simulink model "DPTSpiceModel"  (R2016a)
settings: Solver=FixedStepDiscrete  StartTime=0.0  StopTime=0.55e-6  FixedStep=SampleTime  RelTol=1e-3
values from neighbouring files (symbols this model uses):
  Dbot = 48    [DPTSpiceMFile.m]    (also in LossCalcModelMFile.m = 49)
  DelayBot = 50    [DPTSpiceMFile.m]    (also in LossCalcModelMFile.m)
  DelayTop = 0    [DPTSpiceMFile.m]    (also in LossCalcModelMFile.m)
  Dtop = 48    [DPTSpiceMFile.m]    (also in LossCalcModelMFile.m = 49)
  fsw = 2000e3    (= 2000000)    [DPTSpiceMFile.m]    (also in LossCalcModelMFile.m = 1000000)
  InitialCurrent = LoadCurrent + CurrRipple/2    (= 30.1)    [DPTSpiceMFile.m]
  LoadCurrent = 30    [DPTSpiceMFile.m]
  Rd = 0.0024 + 1e-4    (= 0.0025)    [DPTSpiceMFile.m]    (also in LossCalcModelMFile.m = 2.5e-05; StepResponse.m)
  Rg = 1.5    [DPTSpiceMFile.m]    (also in LossCalcModelMFile.m; StepResponse.m)
  Roff = 2    [DPTSpiceMFile.m]    (also in LossCalcModelMFile.m = 5)
  Ron = 10    [DPTSpiceMFile.m]    (also in LossCalcModelMFile.m = 20)
  Rs = 0.0433 + 1e-4    (= 0.0434)    [DPTSpiceMFile.m]    (also in LossCalcModelMFile.m = 2.5e-05; StepResponse.m)
  Rss = 1e-3    (= 0.001)    [DPTSpiceMFile.m]    (also in StepResponse.m)
  SampleTime = 5e-13    [DPTSpiceMFile.m]    (also in LossCalcModelMFile.m)
  Vdc = 400    [DPTSpiceMFile.m]    (also in LossCalcModelMFile.m)
  VpulseMax = 6    [DPTSpiceMFile.m]    (also in LossCalcModelMFile.m; StepResponse.m)
  VpulseMin = -3    [DPTSpiceMFile.m]    (also in LossCalcModelMFile.m; StepResponse.m)
undefined symbols (not defined in the file or in its folder): DiscIntNeverNeededParam
libraries: elec_lib x50, nesl_utility x34, fl_lib x30, simulink x2
(part 1 of 2)
settings Model: Creator=ugurm  LastModifiedBy=kkfrk
settings OptimizationCC: EfficientMapNaN2IntZero=off
settings HardwareCC: TargetBitPerPointer=64  TargetLongLongMode=on  TargetIntDivRoundTo=Zero  TargetEndianess=LittleEndian  TargetWordSize=64  TargetHWDeviceType=MATLAB Host  ProdEqTarget=off
settings CodeAppCC: MaxIdLength=128
settings GRTTargetCC: GeneratePreprocessorConditionals=Use local settings  CombineOutputUpdateFcns=off  GRTInterface=on

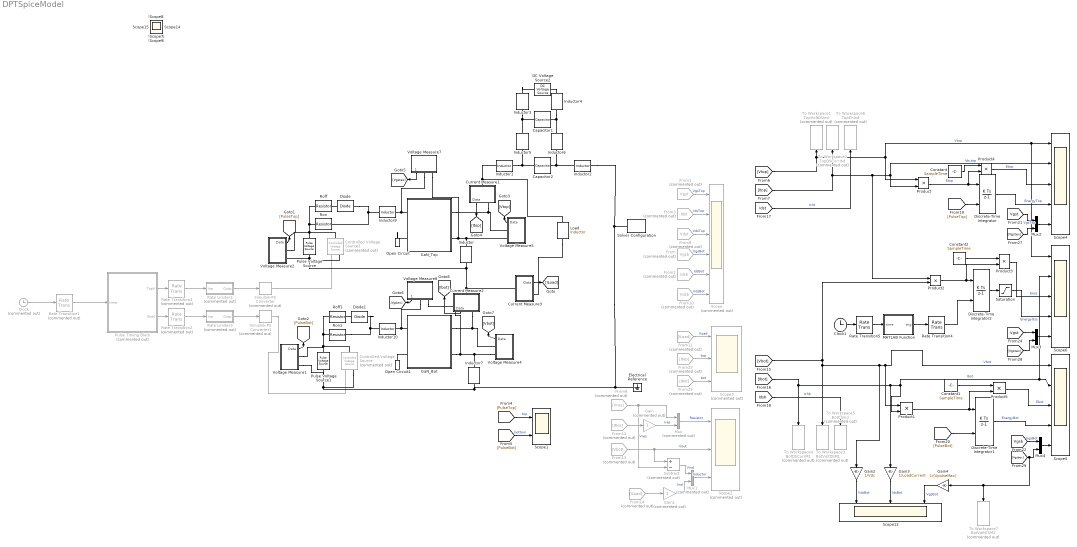
== system DPTSpiceModel ==
  Capacitor1 : elec_lib/Passive Devices/Capacitor  enable_table=0  c=100e-6 F  Cvec=[ 1e-5 1e-6 ] F  Vvec=[ 0 10 ] V  CV_table_symmetry=1  C_tol=5  enable_C_tol=0  tol_distribution=1  nSigma=4  r=1e-6 Ohm  g=0 1/Ohm  initV=Vdc V  enable_operating_limits=0  operating_limit_action=2  max_working_voltage_range=[ -25 25 ] V  power_rating=1 W  enable_faults=0  fault_action=1  Cscale_faulted=100  R_faulted=0.001 Ohm  G_faulted=0 1/Ohm  tau_fault=0.001 s  enable_temporal_fault=0  t_fault=1 s  enable_behavioral_fault=0  max_permissible_voltage_range=[ -100 100 ] V  t_fail_on_voltage=1 s
  Capacitor2 : elec_lib/Passive Devices/Capacitor  enable_table=0  c=2e-6 F  Cvec=[ 1e-5 1e-6 ] F  Vvec=[ 0 10 ] V  CV_table_symmetry=1  C_tol=5  enable_C_tol=0  tol_distribution=1  nSigma=4  r=1e-6 Ohm  g=0 1/Ohm  initV=Vdc V  enable_operating_limits=0  operating_limit_action=2  max_working_voltage_range=[ -25 25 ] V  power_rating=1 W  enable_faults=0  fault_action=1  Cscale_faulted=100  R_faulted=0.001 Ohm  G_faulted=0 1/Ohm  tau_fault=0.001 s  enable_temporal_fault=0  t_fault=1 s  enable_behavioral_fault=0  max_permissible_voltage_range=[ -100 100 ] V  t_fail_on_voltage=1 s
  Clock : Clock  Commented=on
  Clock1 : Clock
  Constant : Constant  Value=SampleTime
  Constant1 : Constant  Value=SampleTime
  Constant2 : Constant  Value=SampleTime
  Controlled Voltage Source : fl_lib/Electrical/Electrical Sources/Controlled Voltage Source  Commented=on
  Controlled Voltage Source1 : fl_lib/Electrical/Electrical Sources/Controlled Voltage Source  Commented=on
  Current Measure1 : Subsystem
  Current Measure2 : Subsystem
  Current Measure3 : Subsystem
  DC Voltage Source2 : elec_lib/Additional Components/SPICE-Compatible Components/Sources/DC Voltage Source  DC=Vdc V
  Diode : elec_lib/Semiconductor Devices/Diode  ModelType=1  Vf=0.3 V  Ron=15e-3 Ohm  Goff=1e-8 S  Rz=0.3 Ohm  Vz=50 V  C_PWL=5 pF  prmExp=1  I12=[ 0.0137 0.545 ] A  V12=[ 0.6 0.7 ] V  I1=0.0137 A  V1=0.6 V  RS=0.01 Ohm  IS=1e-12 A  Tmeas=25 degC  ec=1  BV=Inf V  C_param=1  CJ0=5 pF  VJ=1 V  Mgrad=0.5  Vvec=[ 0.1 10 100 ] V  Cvec=[ 3.5 1 0.4 ] pF  FC=0.5  Q_param=1  Irrm=-7.15 A  iF=4 A  didt=-750 A/us  trr=115 ns  TT=50 ns  tau=100 ns  T_param=1  IS_T2=1.25e-7 A  I1_T2=0.245 A  V1_T2=0.5 V  Tmeas2=125 degC  EG_param=1  EG=1.11 eV  XTI_param=1  XTI=3  dBVdT=0 V/K  Tdevice=25 degC  Rth=[ 0 10 ] K/W  thermal_mass_parameterization=1  thermal_mass=[ 0 1 ] J/K  thermal_time_constant=[ 0 10 ] s  thermal_mass_initial_temperatures=[ 25 25 ] degC
  Diode1 : elec_lib/Semiconductor Devices/Diode  ModelType=1  Vf=0.3 V  Ron=15e-3 Ohm  Goff=1e-8 S  Rz=0.3 Ohm  Vz=50 V  C_PWL=5 pF  prmExp=1  I12=[ 0.0137 0.545 ] A  V12=[ 0.6 0.7 ] V  I1=0.0137 A  V1=0.6 V  RS=0.01 Ohm  IS=1e-12 A  Tmeas=25 degC  ec=1  BV=Inf V  C_param=1  CJ0=5 pF  VJ=1 V  Mgrad=0.5  Vvec=[ 0.1 10 100 ] V  Cvec=[ 3.5 1 0.4 ] pF  FC=0.5  Q_param=1  Irrm=-7.15 A  iF=4 A  didt=-750 A/us  trr=115 ns  TT=50 ns  tau=100 ns  T_param=1  IS_T2=1.25e-7 A  I1_T2=0.245 A  V1_T2=0.5 V  Tmeas2=125 degC  EG_param=1  EG=1.11 eV  XTI_param=1  XTI=3  dBVdT=0 V/K  Tdevice=25 degC  Rth=[ 0 10 ] K/W  thermal_mass_parameterization=1  thermal_mass=[ 0 1 ] J/K  thermal_time_constant=[ 0 10 ] s  thermal_mass_initial_temperatures=[ 25 25 ] degC
  Discrete-Time Integrator : DiscreteIntegrator  ExternalReset=either  InitialConditionSetting=State (most efficient)  SampleTime=-1  ICPrevOutput=DiscIntNeverNeededParam  ICPrevScaledInput=DiscIntNeverNeededParam
  Discrete-Time Integrator1 : DiscreteIntegrator  ExternalReset=either  InitialConditionSetting=State (most efficient)  SampleTime=-1  ICPrevOutput=DiscIntNeverNeededParam  ICPrevScaledInput=DiscIntNeverNeededParam
  Discrete-Time Integrator2 : DiscreteIntegrator  ExternalReset=either  InitialConditionSetting=State (most efficient)  SampleTime=-1  ICPrevOutput=DiscIntNeverNeededParam  ICPrevScaledInput=DiscIntNeverNeededParam
  Electrical Reference : fl_lib/Electrical/Electrical Elements/Electrical Reference
  From : From  Commented=on  GotoTag=Vgsb  TagVisibility=global
  From1 : From  Commented=on  GotoTag=Vgst  TagVisibility=global
  From10 : From  Commented=on  GotoTag=Vdsb  TagVisibility=global
  From11 : From  Commented=on  GotoTag=ILoad
  From12 : From  Commented=on  GotoTag=IRes
  From13 : From  Commented=on  GotoTag=Vbot
  From14 : From  Commented=on  GotoTag=ILoad
  From2 : From  Commented=on  GotoTag=Idsb  TagVisibility=global
  From23 : From  Commented=on  GotoTag=Itop
  From25 : From  Commented=on  GotoTag=Ibot
  From3 : From  Commented=on  GotoTag=Idst  TagVisibility=global
  From8 : From  Commented=on  GotoTag=Vres
  From9 : From  Commented=on  GotoTag=Vdst  TagVisibility=global
  GaN_Bot : Subsystem
  GaN_Top : Subsystem
  Gain : Gain  Commented=on
  Gain1 : Gain  Commented=on
  Gain2 : Gain  Gain=1/Vdc
  Gain3 : Gain  Gain=1/LoadCurrent
  Gain4 : Gain  Gain=1/(VpulseMax)
  Inductor : elec_lib/Passive Devices/Inductor  l=10e-12 H  L_tol=20  enable_L_tol=0  tol_distribution=1  nSigma=4  r=0 Ohm  g=1e-9 1/Ohm  initI=-InitialCurrent A  enable_operating_limits=0  operating_limit_action=2  max_working_current=1 A  power_rating=1 W  enable_faults=0  fault_action=1  lambdaPercent=50  k_faulted=0.9999 Ohm  turnsShort=0  openCct=0  groundShort=0  groundShortG=0 1/Ohm  tau_fault=0.001 s  enable_temporal_fault=0  t_fault=1 s  enable_behavioral_fault=0  max_permissible_voltage=100 V  n_fail_on_voltage=1  max_permissible_current=1 A  t_fail_on_current=1 s
  Inductor1 : elec_lib/Passive Devices/Inductor  l=Ldc H  L_tol=20  enable_L_tol=0  tol_distribution=1  nSigma=4  r=0 Ohm  g=1e-9 1/Ohm  initI=0 A  enable_operating_limits=0  operating_limit_action=1  max_working_current=1 A  power_rating=1 W  enable_faults=0  fault_action=1  lambdaPercent=50  k_faulted=0.9999 Ohm  turnsShort=0  openCct=0  groundShort=0  groundShortG=0 1/Ohm  tau_fault=0.001 s  enable_temporal_fault=0  t_fault=1 s  enable_behavioral_fault=0  max_permissible_voltage=100 V  n_fail_on_voltage=1  max_permissible_current=1 A  t_fail_on_current=1 s
  Inductor10 : elec_lib/Passive Devices/Inductor  l=Lgex H  L_tol=20  enable_L_tol=0  tol_distribution=1  nSigma=4  r=0 Ohm  g=1e-9 1/Ohm  initI=0 A  enable_operating_limits=0  operating_limit_action=1  max_working_current=1 A  power_rating=1 W  enable_faults=0  fault_action=1  lambdaPercent=50  k_faulted=0.9999 Ohm  turnsShort=0  openCct=0  groundShort=0  groundShortG=0 1/Ohm  tau_fault=0.001 s  enable_temporal_fault=0  t_fault=1 s  enable_behavioral_fault=0  max_permissible_voltage=100 V  n_fail_on_voltage=1  max_permissible_current=1 A  t_fail_on_current=1 s
  Inductor2 : elec_lib/Passive Devices/Inductor  l=Ldc H  L_tol=20  enable_L_tol=0  tol_distribution=1  nSigma=4  r=0 Ohm  g=1e-9 1/Ohm  initI=0 A  enable_operating_limits=0  operating_limit_action=1  max_working_current=1 A  power_rating=1 W  enable_faults=0  fault_action=1  lambdaPercent=50  k_faulted=0.9999 Ohm  turnsShort=0  openCct=0  groundShort=0  groundShortG=0 1/Ohm  tau_fault=0.001 s  enable_temporal_fault=0  t_fault=1 s  enable_behavioral_fault=0  max_permissible_voltage=100 V  n_fail_on_voltage=1  max_permissible_current=1 A  t_fail_on_current=1 s
  Inductor3 : elec_lib/Passive Devices/Inductor  l=10e-6 H  L_tol=20  enable_L_tol=0  tol_distribution=1  nSigma=4  r=0 Ohm  g=1e-9 1/Ohm  initI=0 A  enable_operating_limits=0  operating_limit_action=2  max_working_current=1 A  power_rating=1 W  enable_faults=0  fault_action=1  lambdaPercent=50  k_faulted=0.9999 Ohm  turnsShort=0  openCct=0  groundShort=0  groundShortG=0 1/Ohm  tau_fault=0.001 s  enable_temporal_fault=0  t_fault=1 s  enable_behavioral_fault=0  max_permissible_voltage=100 V  n_fail_on_voltage=1  max_permissible_current=1 A  t_fail_on_current=1 s
  Inductor4 : elec_lib/Passive Devices/Inductor  l=10e-6 H  L_tol=20  enable_L_tol=0  tol_distribution=1  nSigma=4  r=0 Ohm  g=1e-9 1/Ohm  initI=0 A  enable_operating_limits=0  operating_limit_action=2  max_working_current=1 A  power_rating=1 W  enable_faults=0  fault_action=1  lambdaPercent=50  k_faulted=0.9999 Ohm  turnsShort=0  openCct=0  groundShort=0  groundShortG=0 1/Ohm  tau_fault=0.001 s  enable_temporal_fault=0  t_fault=1 s  enable_behavioral_fault=0  max_permissible_voltage=100 V  n_fail_on_voltage=1  max_permissible_current=1 A  t_fail_on_current=1 s
  Inductor5 : elec_lib/Passive Devices/Inductor  l=2e-9 H  L_tol=20  enable_L_tol=0  tol_distribution=1  nSigma=4  r=0 Ohm  g=1e-9 1/Ohm  initI=0 A  enable_operating_limits=0  operating_limit_action=2  max_working_current=1 A  power_rating=1 W  enable_faults=0  fault_action=1  lambdaPercent=50  k_faulted=0.9999 Ohm  turnsShort=0  openCct=0  groundShort=0  groundShortG=0 1/Ohm  tau_fault=0.001 s  enable_temporal_fault=0  t_fault=1 s  enable_behavioral_fault=0  max_permissible_voltage=100 V  n_fail_on_voltage=1  max_permissible_current=1 A  t_fail_on_current=1 s
  Inductor6 : elec_lib/Passive Devices/Inductor  l=2e-9 H  L_tol=20  enable_L_tol=0  tol_distribution=1  nSigma=4  r=0 Ohm  g=1e-9 1/Ohm  initI=0 A  enable_operating_limits=0  operating_limit_action=2  max_working_current=1 A  power_rating=1 W  enable_faults=0  fault_action=1  lambdaPercent=50  k_faulted=0.9999 Ohm  turnsShort=0  openCct=0  groundShort=0  groundShortG=0 1/Ohm  tau_fault=0.001 s  enable_temporal_fault=0  t_fault=1 s  enable_behavioral_fault=0  max_permissible_voltage=100 V  n_fail_on_voltage=1  max_permissible_current=1 A  t_fail_on_current=1 s
  Inductor7 : elec_lib/Passive Devices/Inductor  l=10e-12 H  L_tol=20  enable_L_tol=0  tol_distribution=1  nSigma=4  r=0 Ohm  g=1e-9 1/Ohm  initI=0 A  enable_operating_limits=0  operating_limit_action=1  max_working_current=1 A  power_rating=1 W  enable_faults=0  fault_action=1  lambdaPercent=50  k_faulted=0.9999 Ohm  turnsShort=0  openCct=0  groundShort=0  groundShortG=0 1/Ohm  tau_fault=0.001 s  enable_temporal_fault=0  t_fault=1 s  enable_behavioral_fault=0  max_permissible_voltage=100 V  n_fail_on_voltage=1  max_permissible_current=1 A  t_fail_on_current=1 s
  Inductor9 : elec_lib/Passive Devices/Inductor  l=Lgex H  L_tol=20  enable_L_tol=0  tol_distribution=1  nSigma=4  r=0 Ohm  g=1e-9 1/Ohm  initI=0 A  enable_operating_limits=0  operating_limit_action=1  max_working_current=1 A  power_rating=1 W  enable_faults=0  fault_action=1  lambdaPercent=50  k_faulted=0.9999 Ohm  turnsShort=0  openCct=0  groundShort=0  groundShortG=0 1/Ohm  tau_fault=0.001 s  enable_temporal_fault=0  t_fault=1 s  enable_behavioral_fault=0  max_permissible_voltage=100 V  n_fail_on_voltage=1  max_permissible_current=1 A  t_fail_on_current=1 s
  Load : elec_lib/Passive Devices/Inductor  l=Lload H  L_tol=20  enable_L_tol=0  tol_distribution=1  nSigma=4  r=0 Ohm  g=1e-9 1/Ohm  initI=InitialCurrent A  enable_operating_limits=0  operating_limit_action=2  max_working_current=1 A  power_rating=1 W  enable_faults=0  fault_action=1  lambdaPercent=50  k_faulted=0.9999 Ohm  turnsShort=0  openCct=0  groundShort=0  groundShortG=0 1/Ohm  tau_fault=0.001 s  enable_temporal_fault=0  t_fault=1 s  enable_behavioral_fault=0  max_permissible_voltage=100 V  n_fail_on_voltage=1  max_permissible_current=1 A  t_fail_on_current=1 s
  MATLAB Function : MATLAB Function  TreatAsAtomicUnit=on  SystemSampleTime=1e-10
  Mux : Mux  Commented=on  Inputs=2
  Mux1 : Mux  Commented=on  Inputs=2
  Mux2 : Mux  Inputs=2
  Mux3 : Mux  Inputs=2
  Mux4 : Mux  Inputs=2
  Open Circuit : fl_lib/Electrical/Electrical Elements/Open Circuit  v_specify=off  v_priority=None  v=0 V
  Open Circuit1 : fl_lib/Electrical/Electrical Elements/Open Circuit  v_specify=off  v_priority=None  v=0 V
  Product{,1..5} (6 alike) : Product
  Pulse Timing Block : MATLAB Function  Commented=on  TreatAsAtomicUnit=on  SystemSampleTime=1e-9
  Pulse Voltage Source : elec_lib/Additional Components/SPICE-Compatible Components/Sources/Pulse Voltage Source  V1=VpulseMin V  V2=VpulseMax V  TD=DelayTop/(100*fsw) s  TR=1e-9 s  TF=1e-9 s  PW=Dtop/(100*fsw) s  PER=1/fsw s
  Pulse Voltage Source1 : elec_lib/Additional Components/SPICE-Compatible Components/Sources/Pulse Voltage Source  V1=VpulseMin V  V2=VpulseMax V  TD=DelayBot/(100*fsw) s  TR=1e-9 s  TF=1e-9 s  PW=Dbot/(100*fsw) s  PER=1/fsw s
  Rate Limiter2 : Subsystem  Commented=on
  Rate Limiter3 : Subsystem  Commented=on
  Rate Transition1 : RateTransition  Commented=on  OutPortSampleTime=1e-9
  Rate Transition2 : RateTransition  Commented=on  OutPortSampleTime=SampleTime
  Rate Transition3 : RateTransition  Commented=on  OutPortSampleTime=SampleTime
  Rate Transition4 : RateTransition  OutPortSampleTime=SampleTime
  Rate Transition5 : RateTransition  OutPortSampleTime=1e-10
  Roff : elec_lib/Passive Devices/Resistor  R=Roff Ohm  R_tol=5  enable_R_tol=0  tol_distribution=1  nSigma=4  enable_operating_limits=0  operating_limit_action=2  max_working_voltage=100 V  power_rating=1 W  enable_faults=0  fault_action=1  R_faulted=Inf Ohm  enable_temporal_fault=0  t_fault=1 s  enable_behavioral_fault=0  max_permissible_current=1 A  t_fail_on_current=1 s  noise_mode=0  sample_time=0.001 s  repeatability=1  auto_seed=2348838240  user_seed=0  Tdevice=25 degC  alpha=0.00393 1/K  Tmeas=25 degC  thermal_mass=100 J/K  initial_temperature=25 degC  power_derating_T1=70 degC  power_derating_T2=155 degC  operating_temperature_range_vec=[ -50 150 ] degC
  Roff1 : elec_lib/Passive Devices/Resistor  R=Roff Ohm  R_tol=5  enable_R_tol=0  tol_distribution=1  nSigma=4  enable_operating_limits=0  operating_limit_action=2  max_working_voltage=100 V  power_rating=1 W  enable_faults=0  fault_action=1  R_faulted=Inf Ohm  enable_temporal_fault=0  t_fault=1 s  enable_behavioral_fault=0  max_permissible_current=1 A  t_fail_on_current=1 s  noise_mode=0  sample_time=0.001 s  repeatability=1  auto_seed=4112460543  user_seed=0  Tdevice=25 degC  alpha=0.00393 1/K  Tmeas=25 degC  thermal_mass=100 J/K  initial_temperature=25 degC  power_derating_T1=70 degC  power_derating_T2=155 degC  operating_temperature_range_vec=[ -50 150 ] degC
  Ron : elec_lib/Passive Devices/Resistor  R=Ron Ohm  R_tol=5  enable_R_tol=0  tol_distribution=1  nSigma=4  enable_operating_limits=0  operating_limit_action=2  max_working_voltage=100 V  power_rating=1 W  enable_faults=0  fault_action=1  R_faulted=Inf Ohm  enable_temporal_fault=0  t_fault=1 s  enable_behavioral_fault=0  max_permissible_current=1 A  t_fail_on_current=1 s  noise_mode=0  sample_time=0.001 s  repeatability=1  auto_seed=4144164703  user_seed=0  Tdevice=25 degC  alpha=0.00393 1/K  Tmeas=25 degC  thermal_mass=100 J/K  initial_temperature=25 degC  power_derating_T1=70 degC  power_derating_T2=155 degC  operating_temperature_range_vec=[ -50 150 ] degC
  Ron1 : elec_lib/Passive Devices/Resistor  R=Ron Ohm  R_tol=5  enable_R_tol=0  tol_distribution=1  nSigma=4  enable_operating_limits=0  operating_limit_action=2  max_working_voltage=100 V  power_rating=1 W  enable_faults=0  fault_action=1  R_faulted=Inf Ohm  enable_temporal_fault=0  t_fault=1 s  enable_behavioral_fault=0  max_permissible_current=1 A  t_fail_on_current=1 s  noise_mode=0  sample_time=0.001 s  repeatability=1  auto_seed=676943032  user_seed=0  Tdevice=25 degC  alpha=0.00393 1/K  Tmeas=25 degC  thermal_mass=100 J/K  initial_temperature=25 degC  power_derating_T1=70 degC  power_derating_T2=155 degC  operating_temperature_range_vec=[ -50 150 ] degC
  Saturation : Saturate  UpperLimit=100e-6  LowerLimit=0
  Scope : Scope  Commented=on  NumInputPorts=6
  Scope1 : Scope  NumInputPorts=2
  Scope12 : Scope  NumInputPorts=3
  Scope2 : Scope  Commented=on  NumInputPorts=3
  Scope3 : Scope  Commented=on  NumInputPorts=3
  Scope4 : Scope  NumInputPorts=5
  Scope5 : Scope  NumInputPorts=5
  Scope6 : Scope  NumInputPorts=5
  Simulink-PS Converter : nesl_utility/Simulink-PS Converter  Commented=on  PhysicalDomain=network_engine_domain  SubClassName=ps_input  LeftPortType=input  RightPortType=output  PseudoPeriodic=off  Frequencies=[]  NoiseDistribution=none  NoiseParameters=[]  Unit=1  AffineConversion=off  InputFiltering=off  SimscapeFilterOrder=1  InputFilterTimeConstant=0.001  UdotUserProvided=1
  Simulink-PS Converter1 : nesl_utility/Simulink-PS Converter  Commented=on  PhysicalDomain=network_engine_domain  SubClassName=ps_input  LeftPortType=input  RightPortType=output  PseudoPeriodic=off  Frequencies=[]  NoiseDistribution=none  NoiseParameters=[]  Unit=1  AffineConversion=off  InputFiltering=off  SimscapeFilterOrder=1  InputFilterTimeConstant=0.001  UdotUserProvided=1
  Solver Configuration : nesl_utility/Solver Configuration  PhysicalDomain=network_engine_domain  SubClassName=solver  LeftPortType=input  RightPortType=generic  Accelerate=off  Tones=[]  Harmonics=[]  SimulateNoise=off  Profile=off  UseLocalSampling=off  EnableSwitchedLinearOptims=on  FrequencyDomain=off  UseCCode=off  RelTol=0.001  AbsTol=1e-06  MinStep=1e-09  ToWorkspace=off  RevertToSquareIcSolve=off  NumHomotopyIterations=100  PhasorMode=off  PhasorModeNumHarmonics=1  OverrideAbsTol=off  DoDC=off  ResidualTolerance=1e-09  UseLocalSolver=on  LocalSolverChoice=NE_BACKWARD_EULER_ADVANCER  LocalSolverSampleTime=SampleTime  DoFixedCost=on  MaxNonlinIter=3  MaxModeIter=2  LinearAlgebra=Sparse  DelaysMemoryBudget=1024  AutomaticFiltering=on  FilteringTimeConstant=0.001
  Subtract : Sum  Commented=on  Inputs=+-
  To Workspace1 : ToWorkspace  Commented=on  VariableName=TopVoltDSInd  SampleTime=-1
      settings: Save2DSignal=2-D array (concatenate along first dimension)
  To Workspace2 : ToWorkspace  Commented=on  VariableName=TopDSCurrInd  SampleTime=-1
      settings: Save2DSignal=2-D array (concatenate along first dimension)
  To Workspace3 : ToWorkspace  Commented=on  VariableName=BotVoltDSM1  SampleTime=-1
      settings: Save2DSignal=2-D array (concatenate along first dimension)
  To Workspace4 : ToWorkspace  Commented=on  VariableName=BotDSCurrM1  SampleTime=-1
      settings: Save2DSignal=2-D array (concatenate along first dimension)
  To Workspace5 : ToWorkspace  Commented=on  VariableName=BotChInd  SampleTime=-1
      settings: Save2DSignal=2-D array (concatenate along first dimension)
  To Workspace6 : ToWorkspace  Commented=on  VariableName=TopChInd  SampleTime=-1
      settings: Save2DSignal=2-D array (concatenate along first dimension)
  To Workspace7 : ToWorkspace  Commented=on  VariableName=BotVoltGSM1  SampleTime=-1
      settings: Save2DSignal=2-D array (concatenate along first dimension)
  Voltage Measure1 : Subsystem
  Voltage Measure2 : Subsystem
  Voltage Measure4 : Subsystem
  Voltage Measure5 : Subsystem
  Voltage Measure7 : Subsystem
  Voltage Measure8 : Subsystem
  Scope{7..11,13..15} (8 alike) : Scope
  wires:
  Current Measure3/1(Data) -> [ILoad]
  From/1 -> Scope/4  "VgsBot"
  From2/1 -> Scope/5  "IdsBot"
  From3/1 -> Scope/2  "IdsTop"
  From1/1 -> Scope/1  "VgsTop"
  From9/1 -> Scope/3  "VdsTop"
  From10/1 -> Scope/6  "VdsBot"
  From11/1 -> Scope3/1  "Iload"
  [PulseTop] -> Scope1/1  "top"
  [PulseBot] -> Scope1/2  "bottom"
  Voltage Measure2/1(Data) -> [PulseTop]
  Voltage Measure1/1(Data) -> [PulseBot]
  Voltage Measure4/1(Data) -> [Vbot]
  From8/1 -> Mux/1, Subtract/2  "Vres"
  From12/1 -> Gain/1
  Mux/1 -> Scope2/1  "Resistor"
  From13/1 -> Scope2/2, Subtract/1  "Vout"
  Mux1/1 -> Scope2/3  "Inductor"
  From14/1 -> Gain1/1
  Subtract/1 -> Mux1/1  "Vind"
  Gain/1 -> Mux/2  "Ires"
  Gain1/1 -> Mux1/2  "Iind"
  Voltage Measure5/1(Data) -> [Vtop]
  Current Measure1/1(Data) -> [Itop]
  Current Measure2/1(Data) -> [Ibot]
  [Itop] -> Product2/1, Scope4/2, Product/2, To Workspace2/1  "Ids,top"
  [Idsb] -> To Workspace5/1  "Ichb"
  [Ibot] -> To Workspace4/1, Gain3/1, Scope6/2, Scope5/2, Product1/2  "Ibot"
  [Idst] -> To Workspace6/1  "Icht"
  Clock/1 -> Rate Transition1/1
  Rate Transition1/1 -> Pulse Timing Block/1(time)
  Rate Transition2/1 -> Rate Limiter3/1(Inp)
  Rate Transition3/1 -> Rate Limiter2/1(Inp)
  Product/1 -> Product4/2, Discrete-Time Integrator/1  "Etop"
  [PulseTop] -> Discrete-Time Integrator/2
  Product1/1 -> Product5/2, Discrete-Time Integrator1/1
  [PulseBot] -> Discrete-Time Integrator1/2
  [Vtop] -> To Workspace1/1, Scope6/1, Scope4/1, Product/1  "Vtop"
  [Vbot] -> Product2/2, To Workspace3/1, Gain2/1, Scope5/1, Product1/1  "Vbot"
  Pulse Timing Block/1(TopV) -> Rate Transition3/1
  Pulse Timing Block/2(BotV) -> Rate Transition2/1
  Rate Limiter2/1(Outp) -> Simulink-PS Converter/1
  Rate Limiter3/1(Outp) -> Simulink-PS Converter1/1
  Product2/1 -> Product3/2, Discrete-Time Integrator2/1
  Discrete-Time Integrator2/1 -> Saturation/1
  Discrete-Time Integrator/1 -> Scope4/4  "EnergyTop"
  Discrete-Time Integrator1/1 -> Scope5/4  "EnergyBot"
  Saturation/1 -> Scope6/4  "EnergyOss"
  Clock1/1 -> Rate Transition5/1
  MATLAB Function/1(trig) -> Rate Transition4/1
  Rate Transition4/1 -> Discrete-Time Integrator2/2
  Rate Transition5/1 -> MATLAB Function/1(time)
  Product3/1 -> Scope6/3  "Eoss"
  Constant2/1 -> Product3/1
  Product4/1 -> Scope4/3  "Etop"
  Constant/1 -> Product4/1
  Product5/1 -> Scope5/3  "Ebot"
  Constant1/1 -> Product5/1
  From23/1 -> Scope3/2  "top"
  From25/1 -> Scope3/3  "bot"
  Gain2/1 -> Scope12/1  "VdsBot"
  Voltage Measure7/1(Data) -> [Vgstex]
  Voltage Measure8/1(Data) -> [Vgsbex]
  Mux2/1 -> Scope4/5
  [Vgst] -> Mux2/1  "VgsTop"
  [Vgstex] -> Mux2/2
  Mux3/1 -> Scope6/5
  [Vgst] -> Mux3/1
  [Vgstex] -> Mux3/2
  Mux4/1 -> Scope5/5
  [Vgsb] -> Mux4/1  "VgsBot"
  [Vgsbex] -> Gain4/1, To Workspace7/1, Mux4/2
  Gain3/1 -> Scope12/2  "IdsBot"
  Gain4/1 -> Scope12/3  "VgsBot"
  connections:
  Ron/RConn1 -- Voltage Measure2/RConn1 -- Controlled Voltage Source1/LConn1 -- Pulse Voltage Source/LConn1 -- Roff/RConn1
  Ron1/RConn1 -- Controlled Voltage Source/LConn1 -- Pulse Voltage Source1/LConn1 -- Voltage Measure1/RConn1 -- Roff1/RConn1
  Roff/LConn1 -- Diode/RConn1
  Roff1/LConn1 -- Diode1/RConn1
  GaN_Top/RConn1 -- Current Measure1/RConn1 -- Voltage Measure5/RConn1
  GaN_Bot/RConn1 -- Current Measure2/RConn1 -- Voltage Measure4/RConn1
  Simulink-PS Converter/RConn1 -- Controlled Voltage Source1/RConn1
  Simulink-PS Converter1/RConn1 -- Controlled Voltage Source/RConn1
  Diode1/LConn1 -- Ron1/LConn1 -- Inductor10/LConn1
  Capacitor2/RConn1 -- Inductor6/LConn1 -- Inductor2/LConn1
  Inductor5/LConn1 -- Inductor1/RConn1 -- Capacitor2/LConn1
  Inductor5/RConn1 -- Inductor3/LConn1 -- Capacitor1/LConn1
  Capacitor1/RConn1 -- Inductor4/LConn1 -- Inductor6/RConn1
  Inductor3/RConn1 -- DC Voltage Source2/LConn1
  DC Voltage Source2/RConn1 -- Inductor4/RConn1
  Diode/LConn1 -- Inductor9/LConn1 -- Ron/LConn1
  Inductor1/LConn1 -- Load/LConn1 -- Current Measure1/LConn1
  Voltage Measure4/RConn2 -- Inductor7/LConn1 -- GaN_Bot/RConn2 -- Voltage Measure8/RConn2
  Inductor9/RConn1 -- GaN_Top/LConn1 -- Voltage Measure7/RConn1
  Inductor10/RConn1 -- Voltage Measure8/RConn1 -- GaN_Bot/LConn1
  Load/RConn1 -- Current Measure3/RConn1
  Voltage Measure5/RConn2 -- Inductor/LConn1 -- GaN_Top/RConn2 -- Voltage Measure7/RConn2
  Inductor7/RConn1 -- Voltage Measure1/RConn2 -- Pulse Voltage Source1/RConn1 -- Controlled Voltage Source/RConn2 -- Inductor2/RConn1 -- Solver Configuration/RConn1 -- Electrical Reference/LConn1
  Controlled Voltage Source1/RConn2 -- Current Measure3/LConn1 -- Current Measure2/LConn1 -- Inductor/RConn1 -- Pulse Voltage Source/RConn1 -- Voltage Measure2/RConn2
  Open Circuit/LConn1 -- GaN_Top/LConn2
  Open Circuit1/LConn1 -- GaN_Bot/LConn2

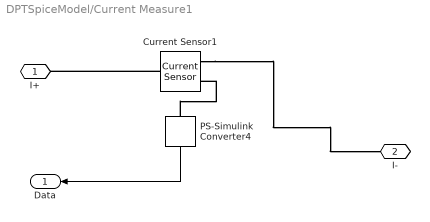
== system DPTSpiceModel/Current Measure1 ==
  Current Sensor1 : fl_lib/Electrical/Electrical Sensors/Current Sensor
  PS-Simulink Converter4 : nesl_utility/PS-Simulink Converter  PhysicalDomain=network_engine_domain  SubClassName=ps_output  LeftPortType=input  RightPortType=output  PseudoPeriodic=off  Frequencies=[]  Unit=1  AffineConversion=off
  I+ : PMIOPort  Port=1  Side=Left
  I- : PMIOPort  Port=2  Side=Right
  Data : Outport
  wires:
  PS-Simulink Converter4/1 -> Data/1
  connections:
  Current Sensor1/RConn2 -- I-/RConn1
  PS-Simulink Converter4/LConn1 -- Current Sensor1/RConn1
  Current Sensor1/LConn1 -- I+/RConn1

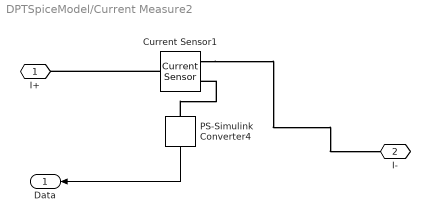
== system DPTSpiceModel/Current Measure2 ==
  Current Sensor1 : fl_lib/Electrical/Electrical Sensors/Current Sensor
  PS-Simulink Converter4 : nesl_utility/PS-Simulink Converter  PhysicalDomain=network_engine_domain  SubClassName=ps_output  LeftPortType=input  RightPortType=output  PseudoPeriodic=off  Frequencies=[]  Unit=1  AffineConversion=off
  I+ : PMIOPort  Port=1  Side=Left
  I- : PMIOPort  Port=2  Side=Right
  Data : Outport
  wires:
  PS-Simulink Converter4/1 -> Data/1
  connections:
  Current Sensor1/RConn2 -- I-/RConn1
  PS-Simulink Converter4/LConn1 -- Current Sensor1/RConn1
  Current Sensor1/LConn1 -- I+/RConn1

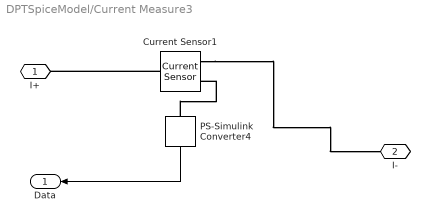
== system DPTSpiceModel/Current Measure3 ==
  Current Sensor1 : fl_lib/Electrical/Electrical Sensors/Current Sensor
  PS-Simulink Converter4 : nesl_utility/PS-Simulink Converter  PhysicalDomain=network_engine_domain  SubClassName=ps_output  LeftPortType=input  RightPortType=output  PseudoPeriodic=off  Frequencies=[]  Unit=1  AffineConversion=off
  I+ : PMIOPort  Port=1  Side=Left
  I- : PMIOPort  Port=2  Side=Right
  Data : Outport
  wires:
  PS-Simulink Converter4/1 -> Data/1
  connections:
  Current Sensor1/LConn1 -- I+/RConn1
  PS-Simulink Converter4/LConn1 -- Current Sensor1/RConn1
  Current Sensor1/RConn2 -- I-/RConn1

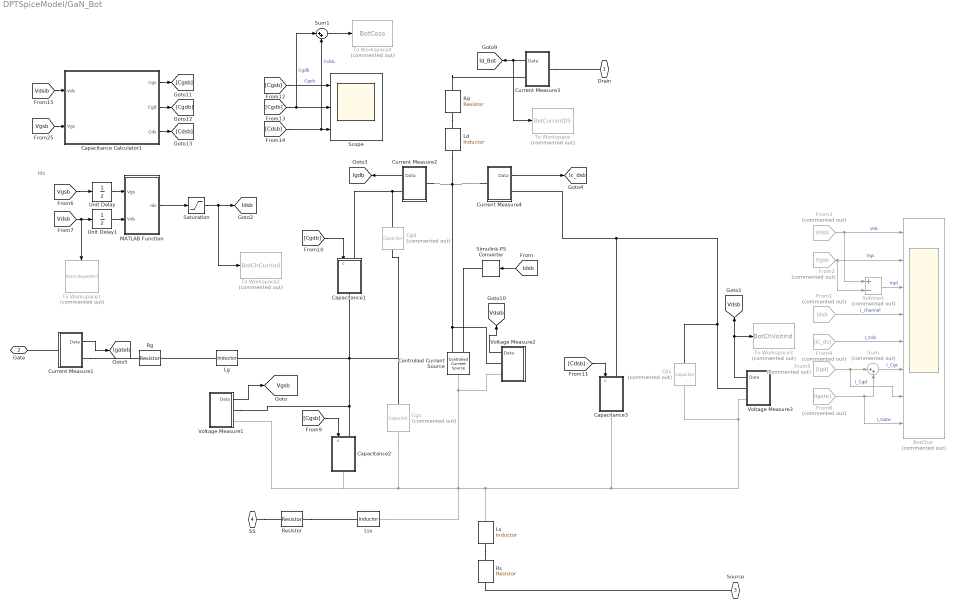
== system DPTSpiceModel/GaN_Bot ==
  note: Ids
  BotChar : Scope  Commented=on  NumInputPorts=8
  Capacitance Calculator1 : Subsystem
  Capacitance1 : Subsystem
  Capacitance2 : Subsystem
  Capacitance3 : Subsystem
  Cds : elec_lib/Passive Devices/Capacitor  Commented=on  enable_table=0  c=Cds F  Cvec=[ 1e-5 1e-6 ] F  Vvec=[ 0 10 ] V  CV_table_symmetry=1  C_tol=5  enable_C_tol=0  tol_distribution=1  nSigma=4  r=1e-6 Ohm  g=0 1/Ohm  initV=0 V  enable_operating_limits=0  operating_limit_action=2  max_working_voltage_range=[ -25 25 ] V  power_rating=1 W  enable_faults=0  fault_action=1  Cscale_faulted=100  R_faulted=0.001 Ohm  G_faulted=0 1/Ohm  tau_fault=0.001 s  enable_temporal_fault=0  t_fault=1 s  enable_behavioral_fault=0  max_permissible_voltage_range=[ -100 100 ] V  t_fail_on_voltage=1 s
  Cgd : elec_lib/Passive Devices/Capacitor  Commented=on  enable_table=0  c=Cgd F  Cvec=[ 1e-5 1e-6 ] F  Vvec=[ 0 10 ] V  CV_table_symmetry=1  C_tol=5  enable_C_tol=0  tol_distribution=1  nSigma=4  r=1e-6 Ohm  g=0 1/Ohm  initV=Vdc - VpulseMin V  enable_operating_limits=0  operating_limit_action=2  max_working_voltage_range=[ -25 25 ] V  power_rating=1 W  enable_faults=0  fault_action=1  Cscale_faulted=100  R_faulted=0.001 Ohm  G_faulted=0 1/Ohm  tau_fault=0.001 s  enable_temporal_fault=0  t_fault=1 s  enable_behavioral_fault=0  max_permissible_voltage_range=[ -100 100 ] V  t_fail_on_voltage=1 s
  Cgs : elec_lib/Passive Devices/Capacitor  Commented=on  enable_table=0  c=Cgs F  Cvec=[ 1e-5 1e-6 ] F  Vvec=[ 0 10 ] V  CV_table_symmetry=1  C_tol=5  enable_C_tol=0  tol_distribution=1  nSigma=4  r=1e-6 Ohm  g=0 1/Ohm  initV=VpulseMax V  enable_operating_limits=0  operating_limit_action=2  max_working_voltage_range=[ -25 25 ] V  power_rating=1 W  enable_faults=0  fault_action=1  Cscale_faulted=100  R_faulted=0.001 Ohm  G_faulted=0 1/Ohm  tau_fault=0.001 s  enable_temporal_fault=0  t_fault=1 s  enable_behavioral_fault=0  max_permissible_voltage_range=[ -100 100 ] V  t_fail_on_voltage=1 s
  Controlled Current Source : fl_lib/Electrical/Electrical Sources/Controlled Current Source
  Current Measure1 : Subsystem
  Current Measure2 : Subsystem
  Current Measure3 : Subsystem
  Current Measure4 : Subsystem
  From1 : From  Commented=on  GotoTag=Idsb  TagVisibility=global
  From2 : From  Commented=on  GotoTag=Vgsb  TagVisibility=global
  From3 : From  Commented=on  GotoTag=Vdsb  TagVisibility=global
  From4 : From  Commented=on  GotoTag=Ic_ds
  From5 : From  Commented=on  GotoTag=Igd
  From8 : From  Commented=on  GotoTag=Igate
  Ld : elec_lib/Passive Devices/Inductor  l=Ld H  L_tol=20  enable_L_tol=0  tol_distribution=1  nSigma=4  r=0 Ohm  g=1e-9 1/Ohm  initI=0 A  enable_operating_limits=0  operating_limit_action=1  max_working_current=1 A  power_rating=1 W  enable_faults=0  fault_action=1  lambdaPercent=50  k_faulted=0.9999 Ohm  turnsShort=0  openCct=0  groundShort=0  groundShortG=0 1/Ohm  tau_fault=0.001 s  enable_temporal_fault=0  t_fault=1 s  enable_behavioral_fault=0  max_permissible_voltage=100 V  n_fail_on_voltage=1  max_permissible_current=1 A  t_fail_on_current=1 s
  "Lg " : elec_lib/Passive Devices/Inductor  l=Lg H  L_tol=20  enable_L_tol=0  tol_distribution=1  nSigma=4  r=0 Ohm  g=1e-9 1/Ohm  initI=0 A  enable_operating_limits=0  operating_limit_action=2  max_working_current=1 A  power_rating=1 W  enable_faults=0  fault_action=1  lambdaPercent=50  k_faulted=0.9999 Ohm  turnsShort=0  openCct=0  groundShort=0  groundShortG=0 1/Ohm  tau_fault=0.001 s  enable_temporal_fault=0  t_fault=1 s  enable_behavioral_fault=0  max_permissible_voltage=100 V  n_fail_on_voltage=1  max_permissible_current=1 A  t_fail_on_current=1 s
  Ls : elec_lib/Passive Devices/Inductor  l=Ls H  L_tol=20  enable_L_tol=0  tol_distribution=1  nSigma=4  r=0 Ohm  g=1e-9 1/Ohm  initI=0 A  enable_operating_limits=0  operating_limit_action=2  max_working_current=1 A  power_rating=1 W  enable_faults=0  fault_action=1  lambdaPercent=50  k_faulted=0.9999 Ohm  turnsShort=0  openCct=0  groundShort=0  groundShortG=0 1/Ohm  tau_fault=0.001 s  enable_temporal_fault=0  t_fault=1 s  enable_behavioral_fault=0  max_permissible_voltage=100 V  n_fail_on_voltage=1  max_permissible_current=1 A  t_fail_on_current=1 s
  Lss : elec_lib/Passive Devices/Inductor  l=Lss H  L_tol=20  enable_L_tol=0  tol_distribution=1  nSigma=4  r=0 Ohm  g=1e-9 1/Ohm  initI=0 A  enable_operating_limits=0  operating_limit_action=1  max_working_current=1 A  power_rating=1 W  enable_faults=0  fault_action=1  lambdaPercent=50  k_faulted=0.9999 Ohm  turnsShort=0  openCct=0  groundShort=0  groundShortG=0 1/Ohm  tau_fault=0.001 s  enable_temporal_fault=0  t_fault=1 s  enable_behavioral_fault=0  max_permissible_voltage=100 V  n_fail_on_voltage=1  max_permissible_current=1 A  t_fail_on_current=1 s
  MATLAB Function : MATLAB Function  TreatAsAtomicUnit=on
  Rd : elec_lib/Passive Devices/Resistor  R=Rd Ohm  R_tol=5  enable_R_tol=0  tol_distribution=1  nSigma=4  enable_operating_limits=0  operating_limit_action=2  max_working_voltage=100 V  power_rating=1 W  enable_faults=0  fault_action=1  R_faulted=Inf Ohm  enable_temporal_fault=0  t_fault=1 s  enable_behavioral_fault=0  max_permissible_current=1 A  t_fail_on_current=1 s  noise_mode=0  sample_time=0.001 s  repeatability=1  auto_seed=3755625184  user_seed=0  Tdevice=25 degC  alpha=0.00393 1/K  Tmeas=25 degC  thermal_mass=100 J/K  initial_temperature=25 degC  power_derating_T1=70 degC  power_derating_T2=155 degC  operating_temperature_range_vec=[ -50 150 ] degC
  Resistor : elec_lib/Passive Devices/Resistor  R=Rss Ohm  R_tol=5  enable_R_tol=0  tol_distribution=1  nSigma=4  enable_operating_limits=0  operating_limit_action=2  max_working_voltage=100 V  power_rating=1 W  enable_faults=0  fault_action=1  R_faulted=Inf Ohm  enable_temporal_fault=0  t_fault=1 s  enable_behavioral_fault=0  max_permissible_current=1 A  t_fail_on_current=1 s  noise_mode=0  sample_time=0.001 s  repeatability=1  auto_seed=5602712  user_seed=0  Tdevice=25 degC  alpha=0.00393 1/K  Tmeas=25 degC  thermal_mass=100 J/K  initial_temperature=25 degC  power_derating_T1=70 degC  power_derating_T2=155 degC  operating_temperature_range_vec=[ -50 150 ] degC
  Rg : elec_lib/Passive Devices/Resistor  R=Rg Ohm  R_tol=5  enable_R_tol=0  tol_distribution=1  nSigma=4  enable_operating_limits=0  operating_limit_action=2  max_working_voltage=100 V  power_rating=1 W  enable_faults=0  fault_action=1  R_faulted=Inf Ohm  enable_temporal_fault=0  t_fault=1 s  enable_behavioral_fault=0  max_permissible_current=1 A  t_fail_on_current=1 s  noise_mode=0  sample_time=0.001 s  repeatability=1  auto_seed=3890346746  user_seed=0  Tdevice=25 degC  alpha=0.00393 1/K  Tmeas=25 degC  thermal_mass=100 J/K  initial_temperature=25 degC  power_derating_T1=70 degC  power_derating_T2=155 degC  operating_temperature_range_vec=[ -50 150 ] degC
  Rs : elec_lib/Passive Devices/Resistor  R=Rs Ohm  R_tol=5  enable_R_tol=0  tol_distribution=1  nSigma=4  enable_operating_limits=0  operating_limit_action=2  max_working_voltage=100 V  power_rating=1 W  enable_faults=0  fault_action=1  R_faulted=Inf Ohm  enable_temporal_fault=0  t_fault=1 s  enable_behavioral_fault=0  max_permissible_current=1 A  t_fail_on_current=1 s  noise_mode=0  sample_time=0.001 s  repeatability=1  auto_seed=466632178  user_seed=0  Tdevice=25 degC  alpha=0.00393 1/K  Tmeas=25 degC  thermal_mass=100 J/K  initial_temperature=25 degC  power_derating_T1=70 degC  power_derating_T2=155 degC  operating_temperature_range_vec=[ -50 150 ] degC
  Saturation : Saturate  UpperLimit=200  LowerLimit=-200
  Scope : Scope  NumInputPorts=3
  Simulink-PS Converter : nesl_utility/Simulink-PS Converter  PhysicalDomain=network_engine_domain  SubClassName=ps_input  LeftPortType=input  RightPortType=output  PseudoPeriodic=off  Frequencies=[]  NoiseDistribution=none  NoiseParameters=[]  Unit=1  AffineConversion=off  InputFiltering=off  SimscapeFilterOrder=1  InputFilterTimeConstant=0.001  UdotUserProvided=1
  Subtract : Sum  Commented=on  Inputs=+-
  Sum : Sum  Commented=on  Inputs=|++
  Sum1 : Sum  Inputs=|++
  To Workspace : ToWorkspace  Commented=on  VariableName=BotCurrentDS  SampleTime=-1
      settings: Save2DSignal=2-D array (concatenate along first dimension)
  To Workspace1 : ToWorkspace  Commented=on  VariableName=BotVoltageDSInd  SampleTime=-1
      settings: Save2DSignal=2-D array (concatenate along first dimension)
  To Workspace2 : ToWorkspace  Commented=on  VariableName=BotChCurrInd  SampleTime=-1
      settings: Save2DSignal=2-D array (concatenate along first dimension)
  To Workspace3 : ToWorkspace  Commented=on  VariableName=BotChVoltInd  SampleTime=-1
      settings: Save2DSignal=2-D array (concatenate along first dimension)
  To Workspace4 : ToWorkspace  Commented=on  VariableName=BotCoss  SampleTime=-1
      settings: Save2DSignal=2-D array (concatenate along first dimension)
  Unit Delay : UnitDelay  SampleTime=-1
  Unit Delay1 : UnitDelay  SampleTime=-1
  Voltage Measure1 : Subsystem
  Voltage Measure2 : Subsystem
  Voltage Measure3 : Subsystem
  Drain : PMIOPort  Port=1  Side=Right
  Gate : PMIOPort  Port=2  Side=Left
  Source : PMIOPort  Port=3  Side=Right
  SS : PMIOPort  Port=4  Side=Left
  tag scope: Ic_dsb=global, Id_Bot=global, Idsb=global, Igateb=global, Igdb=global, Vdsb=global, Vdsib=global, Vgsb=global
  wires:
  Voltage Measure1/1(Data) -> [Vgsb]
  [Vdsb] -> Unit Delay1/1, To Workspace1/1
  Unit Delay/1 -> MATLAB Function/1(Vgs)
  MATLAB Function/1(Ids) -> Saturation/1
  [Vgsb] -> Unit Delay/1
  [Idsb] -> Simulink-PS Converter/1
  From2/1 -> BotChar/2, Subtract/2  "Vgs"
  From3/1 -> BotChar/1, Subtract/1  "Vds"
  From1/1 -> BotChar/4  "I_channel"
  Subtract/1 -> BotChar/3  "Vgd"
  From4/1 -> BotChar/5  "I_Cds"
  From5/1 -> BotChar/7, Sum/1  "I_Cgd"
  From8/1 -> BotChar/8, Sum/2  "I_Gate"
  Current Measure2/1(Data) -> [Igdb]
  Current Measure4/1(Data) -> [Ic_dsb]
  Sum/1 -> BotChar/6  "I_Cgs"
  Current Measure1/1(Data) -> [Igateb]
  Voltage Measure3/1(Data) -> To Workspace3/1, [Vdsb]
  [Cgsb] -> Capacitance2/1(c)
  [Cgdb] -> Capacitance1/1(c)
  [Cdsb] -> Capacitance3/1(c)
  [Cgsb] -> Scope/1  "Cgsb"
  [Cgdb] -> Sum1/1, Scope/2  "Cgdb"
  [Cdsb] -> Sum1/2, Scope/3  "Cdsb"
  Current Measure3/1(Data) -> To Workspace/1, [Id_Bot]
  Unit Delay1/1 -> MATLAB Function/2(Vds)
  Voltage Measure2/1(Data) -> [Vdsib]
  Saturation/1 -> [Idsb], To Workspace2/1
  [Vdsib] -> Capacitance Calculator1/1(Vds)
  Capacitance Calculator1/1(Cgs) -> [Cgsb]
  Capacitance Calculator1/2(Cgd) -> [Cgdb]
  Capacitance Calculator1/3(Cds) -> [Cdsb]
  [Vgsb] -> Capacitance Calculator1/2(Vgs)
  Sum1/1 -> To Workspace4/1
  connections:
  Simulink-PS Converter/RConn1 -- Controlled Current Source/RConn1
  Current Measure1/LConn1 -- Gate/RConn1
  Voltage Measure3/RConn1 -- Cds/LConn1 -- Capacitance3/LConn1 -- Current Measure4/RConn1
  Current Measure1/RConn1 -- Rg/RConn1
  Capacitance1/LConn1 -- Cgd/LConn1 -- Current Measure2/RConn1
  Current Measure3/LConn1 -- Drain/RConn1
  Capacitance2/LConn1 -- Voltage Measure1/RConn1 -- "Lg "/RConn1 -- Cgd/RConn1 -- Cgs/LConn1 -- Capacitance1/RConn1
  Controlled Current Source/RConn2 -- Voltage Measure2/RConn1 -- Ld/RConn1 -- Current Measure2/LConn1 -- Current Measure4/LConn1
  SS/RConn1 -- Resistor/LConn1
  Cds/RConn1 -- Capacitance3/RConn1 -- Ls/LConn1 -- Lss/RConn1 -- Controlled Current Source/LConn1 -- Voltage Measure2/RConn2 -- Voltage Measure1/RConn2 -- Capacitance2/RConn1 -- Cgs/RConn1 -- Voltage Measure3/RConn2
  Rs/RConn1 -- Source/RConn1
  Rd/LConn1 -- Current Measure3/RConn1
  Resistor/RConn1 -- Lss/LConn1
  Rd/RConn1 -- Ld/LConn1
  "Lg "/LConn1 -- Rg/LConn1
  Ls/RConn1 -- Rs/LConn1
